simulink model "q_two_complete"  (R2019b)
settings: Solver=VariableStepAuto  StartTime=0.0  StopTime=0.05  RelTol=1e-3
values from neighbouring files (symbols this model uses):
  A1 = [(-Ra/La) ((-ka*ia)/La); ((ka*ia)/J) (-B/J)]    [ex2.m]    (also in ex3.m = [(-Ra/La) ((-ka*ia)/La); (ka*ia)/J -(B/J)])
  B1 = [(1/La) 0; 0 (-1/J)]    [ex2.m]    (also in ex3.m)
  C1 = [1 0;0 1]    [ex2.m]    (also in ex3.m)
  D1 = [0 0;0 0]    [ex2.m]    (also in ex3.m)
  k = place(open_A1, open_B1, p2)    [ex2.m]
settings Model: Creator=kecy6rkk  LastModifiedBy=rafek
settings SFSimCC: CustomCodeUndefinedFunction=UseInterfaceOnly

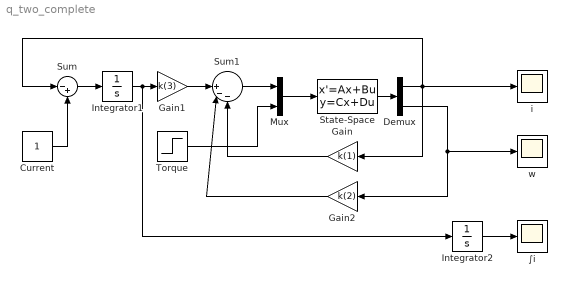
== system q_two_complete ==
  " ∫i" : Scope
  Current : Constant
  Demux : Demux  Outputs=2
  Gain : Gain  Gain=k(1)
  Gain1 : Gain  Gain=k(3)
  Gain2 : Gain  Gain=k(2)
  Integrator1 : Integrator
  Integrator2 : Integrator
  Mux : Mux  Inputs=2
  State-Space : StateSpace  A=A1  B=B1  C=C1  D=D1  InitialCondition=0
  Sum : Sum  Inputs=|-+
  Sum1 : Sum  Inputs=||+--
  Torque : Step  Time=0  After=75  SampleTime=0
  i : Scope
  w : Scope
  wires:
  State-Space/1 -> Demux/1
  Demux/1 -> Gain/1, Sum/1, i/1
  Demux/2 -> Gain2/1, w/1
  Current/1 -> Sum/2
  Integrator1/1 -> Integrator2/1, Gain1/1
  Gain/1 -> Sum1/3
  Gain2/1 -> Sum1/2
  Sum/1 -> Integrator1/1
  Gain1/1 -> Sum1/1
  Sum1/1 -> Mux/1
  Mux/1 -> State-Space/1
  Torque/1 -> Mux/2
  Integrator2/1 -> " ∫i"/1
